simulink subsystem "Reductor"  (R2023a)
settings: Solver=VariableStepAuto  StartTime=0.0  StopTime=10.0  RelTol=1e-3
model mask{J=0, i=0}
  mask prompts: J "Reductor inertia"; i "Reductor ratio"
settings Model: Creator=ycheb  LastModifiedBy=ycheb

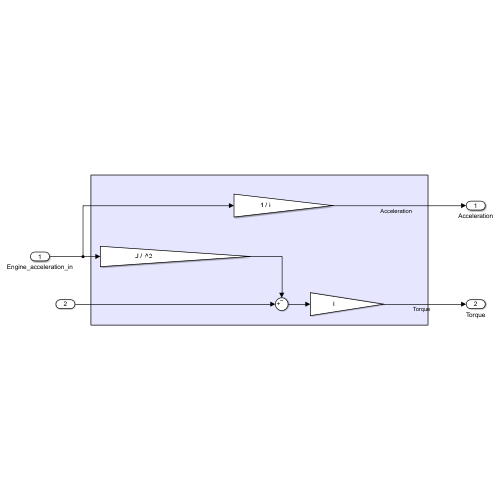
[thumbnail: Simulink's stored preview of the top-level diagram]
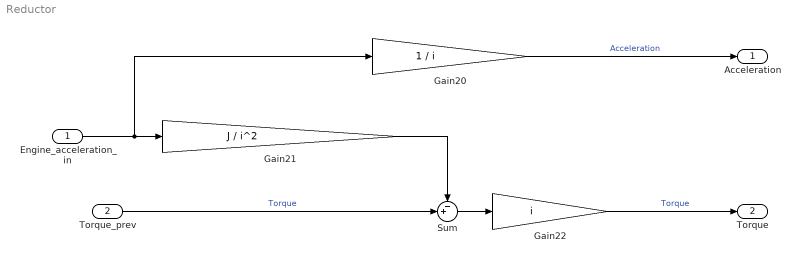
== system Reductor ==
  Engine_acceleration_in : Inport
  Torque_prev : Inport  Port=2
  Gain20 : Gain  Gain=1 / i
  Gain21 : Gain  Gain=J / i^2
  Gain22 : Gain  Gain=i
  Sum : Sum  Inputs=-+|
  Acceleration : Outport
  Torque : Outport  Port=2
  wires:
  Gain20/1 -> Acceleration/1  "Acceleration"
  Gain21/1 -> Sum/1
  Sum/1 -> Gain22/1
  Engine_acceleration_in/1 -> Gain21/1, Gain20/1
  Gain22/1 -> Torque/1  "Torque"
  Torque_prev/1 -> Sum/2  "Torque"
